simulink model "Aula07_ex01"  (Simulink 8.2)
settings: Solver=ode45  StartTime=0.0  StopTime=0.0250  RelTol=1e-3
settings Model: Creator=Andréa  LastModifiedBy=Andréa
settings SimEventsCC: propDiagAttribOutput=1  propDiagFcnCallOutput=1  propDiagStatOutput=0  propPreventDuplicateEvents=0
settings ConfigurationSet: Description=SimMechanics 2G

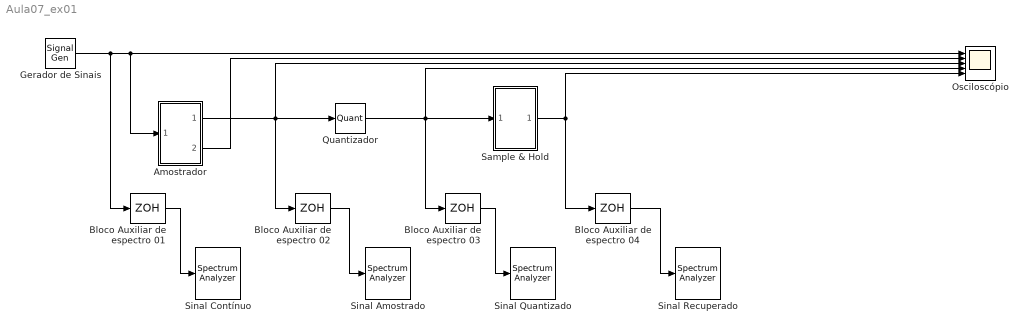
== system Aula07_ex01 ==
  Amostrador : Subsystem
  Bloco Auxiliar de espectro 01 : ZeroOrderHold  SampleTime=1/(6*8000)
  Bloco Auxiliar de espectro 02 : ZeroOrderHold  SampleTime=1/(6*8000)
  Bloco Auxiliar de espectro 03 : ZeroOrderHold  SampleTime=1/(6*8000)
  Bloco Auxiliar de espectro 04 : ZeroOrderHold  SampleTime=1/(6*8000)
  Gerador de Sinais : SignalGenerator  Frequency=500
  Osciloscópio : Scope  NumInputPorts=5
      settings: YMin=-1~-1~-1~-1~-1  YMax=1~1~1~1~1  SampleInput=on  SampleTime=0.00000001
  Quantizador : Quantizer  QuantizationInterval=0.25
  Sample & Hold : Subsystem
  Sinal Amostrado : SpectrumAnalyzer  ScopeSpecification=DataTag0
      settings: CopyFcn=scopeextensions.ScopeBlock.onCoreBlockCopy(gcbh);  DeleteFcn=scopeextensions.ScopeBlock.callback(gcbh, 'onBlockDelete');  PreSaveFcn=scopeextensions.ScopeBlock.callback(gcbh, 'onModelSave');  NameChangeFcn=scopeextensions.ScopeBlock.callback(gcbh, 'onBlockRename');  DestroyFcn=scopeextensions.ScopeBlock.onBlockDestroy(gcbh)  CloseFcn=scopeextensions.ScopeBlock.callback(gcbh, 'onBlockClose');  PreDeleteFcn=scopeextensions.ScopeBlock.callback(gcbh, 'onBlockPreDelete');
  Sinal Contínuo : SpectrumAnalyzer  ScopeSpecification=DataTag1
      settings: CopyFcn=scopeextensions.ScopeBlock.onCoreBlockCopy(gcbh);  DeleteFcn=scopeextensions.ScopeBlock.callback(gcbh, 'onBlockDelete');  PreSaveFcn=scopeextensions.ScopeBlock.callback(gcbh, 'onModelSave');  NameChangeFcn=scopeextensions.ScopeBlock.callback(gcbh, 'onBlockRename');  DestroyFcn=scopeextensions.ScopeBlock.onBlockDestroy(gcbh)  CloseFcn=scopeextensions.ScopeBlock.callback(gcbh, 'onBlockClose');  PreDeleteFcn=scopeextensions.ScopeBlock.callback(gcbh, 'onBlockPreDelete');
  Sinal Quantizado : SpectrumAnalyzer  ScopeSpecification=DataTag2
      settings: CopyFcn=scopeextensions.ScopeBlock.onCoreBlockCopy(gcbh);  DeleteFcn=scopeextensions.ScopeBlock.callback(gcbh, 'onBlockDelete');  PreSaveFcn=scopeextensions.ScopeBlock.callback(gcbh, 'onModelSave');  NameChangeFcn=scopeextensions.ScopeBlock.callback(gcbh, 'onBlockRename');  DestroyFcn=scopeextensions.ScopeBlock.onBlockDestroy(gcbh)  CloseFcn=scopeextensions.ScopeBlock.callback(gcbh, 'onBlockClose');  PreDeleteFcn=scopeextensions.ScopeBlock.callback(gcbh, 'onBlockPreDelete');
  Sinal Recuperado : SpectrumAnalyzer  ScopeSpecification=DataTag3
      settings: CopyFcn=scopeextensions.ScopeBlock.onCoreBlockCopy(gcbh);  DeleteFcn=scopeextensions.ScopeBlock.callback(gcbh, 'onBlockDelete');  PreSaveFcn=scopeextensions.ScopeBlock.callback(gcbh, 'onModelSave');  NameChangeFcn=scopeextensions.ScopeBlock.callback(gcbh, 'onBlockRename');  DestroyFcn=scopeextensions.ScopeBlock.onBlockDestroy(gcbh)  CloseFcn=scopeextensions.ScopeBlock.callback(gcbh, 'onBlockClose');  PreDeleteFcn=scopeextensions.ScopeBlock.callback(gcbh, 'onBlockPreDelete');
  wires:
  Gerador de Sinais/1 -> Bloco Auxiliar de espectro 01/1, Osciloscópio/1, Amostrador/1(In1)
  Amostrador/1(Out1) -> Bloco Auxiliar de espectro 02/1, Quantizador/1, Osciloscópio/3
  Quantizador/1 -> Bloco Auxiliar de espectro 03/1, Sample & Hold/1(In1), Osciloscópio/4
  Sample & Hold/1(Out1) -> Bloco Auxiliar de espectro 04/1, Osciloscópio/5
  Amostrador/2(Out2) -> Osciloscópio/2
  Bloco Auxiliar de espectro 01/1 -> Sinal Contínuo/1
  Bloco Auxiliar de espectro 02/1 -> Sinal Amostrado/1
  Bloco Auxiliar de espectro 03/1 -> Sinal Quantizado/1
  Bloco Auxiliar de espectro 04/1 -> Sinal Recuperado/1

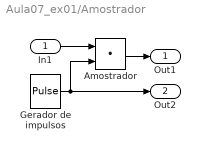
== system Aula07_ex01/Amostrador ==
  In1 : Inport
  Amostrador : DotProduct  InputSameDT=on  OutDataTypeStr=Inherit: Inherit via internal rule
  Gerador de impulsos : DiscretePulseGenerator  PulseType=Time based  Period=1.25e-4
  Out1 : Outport
  Out2 : Outport  Port=2
  wires:
  Gerador de impulsos/1 -> Out2/1, Amostrador/2
  In1/1 -> Amostrador/1
  Amostrador/1 -> Out1/1

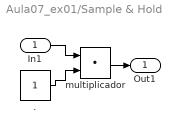
== system Aula07_ex01/Sample & Hold ==
  In1 : Inport
  . : Constant
  multiplicador : DotProduct  SampleTime=1.25e-4  InputSameDT=on  OutDataTypeStr=Inherit: Inherit via internal rule
  Out1 : Outport
  wires:
  In1/1 -> multiplicador/1
  multiplicador/1 -> Out1/1
  ./1 -> multiplicador/2
